simulink subsystem "AngleSensor"  (R2020b)
settings: Solver=VariableStepAuto  StartTime=0.0  StopTime=10.0  RelTol=1e-3
libraries: nesl_utility x3, sm_lib x2
settings Model: Creator=PaulWintz  LastModifiedBy=PaulWintz

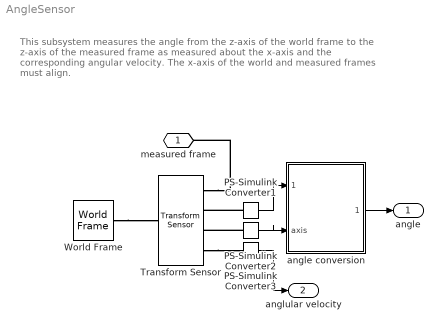
== system AngleSensor ==
  note: This subsystem measures the angle from the z-axis of the
      | world frame to the z-axis of the measured frame as
      | measured about the x-axis and the corresponding angular
      | velocity. The x-axis of the world and
      | measured frames must align.
  PS-Simulink Converter1 : nesl_utility/PS-Simulink Converter  PhysicalDomain=network_engine_domain  SubClassName=ps_output  LeftPortType=input  RightPortType=output  PseudoPeriodic=off  Frequencies=[]  Unit=inherit  AffineConversion=off
  PS-Simulink Converter2 : nesl_utility/PS-Simulink Converter  PhysicalDomain=network_engine_domain  SubClassName=ps_output  LeftPortType=input  RightPortType=output  PseudoPeriodic=off  Frequencies=[]  Unit=inherit  AffineConversion=off
  PS-Simulink Converter3 : nesl_utility/PS-Simulink Converter  PhysicalDomain=network_engine_domain  SubClassName=ps_output  LeftPortType=input  RightPortType=output  PseudoPeriodic=off  Frequencies=[]  Unit=inherit  AffineConversion=off
  Transform Sensor : sm_lib/Frames and Transforms/Transform Sensor  MeasurementFrame=World  SenseAngle=on  SenseAxis=on  SenseAngle1=off  SenseAngle2=off  SenseAngle3=off  SenseQ=off  SenseR=off  SenseOmegaX=on  SenseOmegaY=off  SenseOmegaZ=off  SenseOmega1=off  SenseOmega2=off  SenseOmega3=off  SenseQDot=off  SenseRDot=off  SenseAlphaX=off  SenseAlphaY=off  SenseAlphaZ=off  SenseAlpha1=off  SenseAlpha2=off  SenseAlpha3=off  SenseQDDot=off  SenseRDDot=off  SenseX=off  SenseY=off  SenseZ=off  SenseRad=off  SenseAzim=off  SenseDist=off  SenseInc=off  SenseXDot=off  SenseYDot=off  SenseZDot=off  SenseRadDot=off  SenseAzimDot=off  SenseDistDot=off  SenseIncDot=off  SenseXDDot=off  SenseYDDot=off  SenseZDDot=off  SenseRadDDot=off  SenseAzimDDot=off  SenseDistDDot=off  SenseIncDDot=off
  World Frame : sm_lib/Frames and Transforms/World Frame
  angle conversion : MATLAB Function  TreatAsAtomicUnit=on
  measured frame : PMIOPort  Side=Left
  angle : Outport  PortDimensions=1
  anglular velocity : Outport  Port=2  PortDimensions=1
  wires:
  PS-Simulink Converter1/1 -> angle conversion/1(angle_in)
  angle conversion/1(angle_out) -> angle/1
  PS-Simulink Converter2/1 -> angle conversion/2(axis)
  PS-Simulink Converter3/1 -> anglular velocity/1
  connections:
  Transform Sensor/RConn1 -- measured frame/RConn1
  PS-Simulink Converter1/LConn1 -- Transform Sensor/RConn2
  PS-Simulink Converter2/LConn1 -- Transform Sensor/RConn3
  World Frame/RConn1 -- Transform Sensor/LConn1
  Transform Sensor/RConn4 -- PS-Simulink Converter3/LConn1

== matlab function AngleSensor/angle conversion ==
  data: angle_in input; angle_out output; axis input
function angle_out = angle_about_x(angle_in, axis)
% For a rotation that is purely about the x-axis, this function takes the
% "angle" and "axis" outputs of the transform sensor and returns the
% angle rotated about the x-axis. The reason this is needed is that the
% transform sensor sometimes returns the -x axis so we must switch the sign
% of the rotation. 

if abs(angle_in) < 1e-4
    angle_out = angle_in;
    return
end

assert(abs(axis(1)) == 1, "axis or rotation is not in x direction. angle=%f, axis=(%f, %f, %f)", angle_in, axis(1), axis(2), axis(3));

angle_out = angle_in * axis(1);
